simulink model "tanque"  (R2020a)
settings: Solver=VariableStepAuto  StartTime=0.0  StopTime=20  RelTol=1e-3
undefined symbols (not defined in the file or in its folder): e0, ef, h0
settings Model: Creator=a1  LastModifiedBy=a1

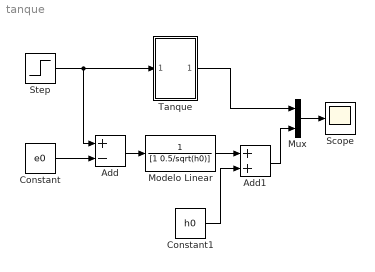
== system tanque ==
  Add : Sum  Inputs=+-
  Add1 : Sum
  Constant : Constant  Value=e0
  Constant1 : Constant  Value=h0
  "Modelo Linear " : TransferFcn  Denominator=[1 0.5/sqrt(h0)]
  Mux : Mux  Inputs=2
  Scope : Scope
  Step : Step  Before=e0  After=ef  SampleTime=0
  Tanque : Subsystem
  wires:
  Step/1 -> Add/1, Tanque/1(e(t))
  Tanque/1(h(t)) -> Mux/1
  Mux/1 -> Scope/1
  Add/1 -> "Modelo Linear "/1
  Constant/1 -> Add/2
  "Modelo Linear "/1 -> Add1/1
  Add1/1 -> Mux/2
  Constant1/1 -> Add1/2

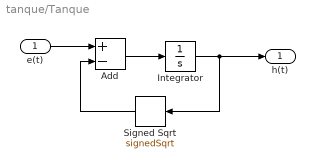
== system tanque/Tanque ==
  e(t) : Inport
  Add : Sum  Inputs=+-
  Integrator : Integrator  InitialCondition=h0
  Signed Sqrt : Sqrt  Operator=signedSqrt  OutputSignalType=real  SaturateOnIntegerOverflow=on
  h(t) : Outport
  wires:
  e(t)/1 -> Add/1
  Signed Sqrt/1 -> Add/2
  Add/1 -> Integrator/1
  Integrator/1 -> h(t)/1, Signed Sqrt/1
